simulink model "c28069_B2Bcontrol_hbT"  (R2018b)
settings: Solver=ode4  StartTime=0.0  StopTime=inf  FixedStep=100e-6*0+0.0001*0+Ts/4  RelTol=1e-3
values from neighbouring files (symbols this model uses):
  Ts = Tsw    (= 3.33333333333e-05)    [data_init_B2B.m]
undefined symbols (not defined in the file or in its folder): serial
libraries: instrumentlib x2
settings Model: Creator=matti  LastModifiedBy=matti
settings DataIOCC: ReturnWorkspaceOutputs=on
settings HardwareCC: ProdBitPerPointer=32  ProdBitPerSizeT=32  ProdBitPerPtrDiffT=32  ProdWordSize=32  ProdHWDeviceType=Intel->x86-32 (Windows32)
settings SFSimCC: SimUseLocalCustomCode=off
settings RTWCC: RTWUseLocalCustomCode=off
settings CodeAppCC: StateflowObjectComments=on
settings SimscapeCC: SimscapeNormalizeSystem=off

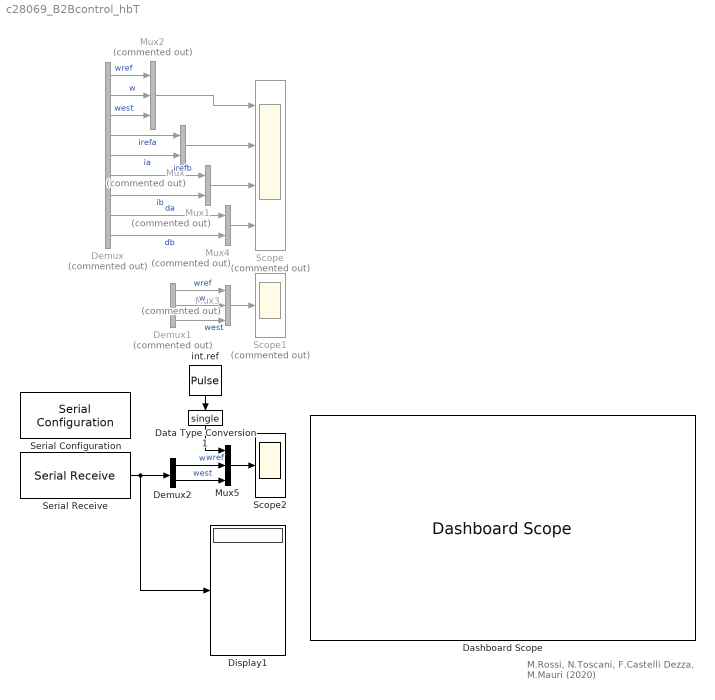
== system c28069_B2Bcontrol_hbT ==
  note: M.Rossi, N.Toscani, F.Castelli Dezza, M.Mauri (2020)
  Dashboard Scope : DashboardScope  WebBlockId=52  TimeSpan=30  Ymin=0  Ymax=150
  Data Type Conversion1 : DataTypeConversion  OutDataTypeStr=single
  Demux : Demux  Commented=on  Outputs=9
  Demux1 : Demux  Commented=on  Outputs=3
  Demux2 : Demux  Outputs=2
  Display1 : Display
  Mux : Mux  Commented=on  Inputs=2
  Mux1 : Mux  Commented=on  Inputs=2
  Mux2 : Mux  Commented=on  Inputs=3
  Mux3 : Mux  Commented=on  Inputs=3
  Mux4 : Mux  Commented=on  Inputs=2
  Mux5 : Mux  Inputs=3
  Scope : Scope  Commented=on  NumInputPorts=4
  Scope1 : Scope  Commented=on
  Scope2 : Scope
  Serial Configuration : instrumentlib/Serial Configuration  Priority=-200000  ComPortMenu=<Please select a port...>  ComPort=COM10  ObjConstructor=serial('COM10');  BaudRate=115200  DataBits=8  Parity=none  StopBits=1  FlowControl=none  Timeout=10  ByteOrder=LittleEndian
  Serial Receive : instrumentlib/Serial Receive  ComPortMenu=<Please select a port...>  ComPort=COM10  ObjConstructor=serial('COM10');  Terminator=<none>  DataSize="[1  2]"  DataType=single  EnableBlockingMode=on  ActionDataUnavailable=Output last received value  CustomValue=0  SampleTime=0.01
  int.ref : DiscretePulseGenerator  Amplitude=100  Period=120000*2  PulseWidth=120000  SampleTime=Ts
  wires:
  Demux/1 -> Mux2/1  "wref"
  Mux/1 -> Scope/2
  Demux/4 -> Mux/1  "irefa"
  Demux/2 -> Mux2/2  "w"
  Mux2/1 -> Scope/1
  Serial Receive/1 -> Display1/1, Demux2/1
  Demux1/2 -> Mux3/2  "w"
  Mux3/1 -> Scope1/1
  int.ref/1 -> Data Type Conversion1/1
  Demux1/3 -> Mux3/3  "west"
  Demux/3 -> Mux2/3  "west"
  Demux/5 -> Mux/2  "ia"
  Demux/6 -> Mux1/1  "irefb"
  Demux/7 -> Mux1/2  "ib"
  Demux/8 -> Mux4/1  "da"
  Demux/9 -> Mux4/2  "db"
  Mux1/1 -> Scope/3
  Mux4/1 -> Scope/4
  Demux1/1 -> Mux3/1  "wref"
  Demux2/2 -> Mux5/3  "west"
  Mux5/1 -> Scope2/1
  Demux2/1 -> Mux5/2  "w"
  Data Type Conversion1/1 -> Mux5/1  "wref"
